simulink model "dc_motor"  (R2015a)
settings: Solver=ode45  StartTime=0.0  StopTime=0.3  RelTol=1e-3
values from neighbouring files (symbols this model uses):
  j = 0.575/1000    (= 0.000575)    [motor_a2b_param.m]    (also in motor_param.m = 0.02)
  k = 0.93    [motor_a2b_param.m]    (also in motor_param.m = 0.796; para.m = 0.5)
  la = 25/1000    (= 0.025)    [motor_a2b_param.m]    (also in motor_param.m = 0.01)
  ra = 7.8    [motor_a2b_param.m]    (also in motor_param.m = 0.78)
libraries: powerlib x5
settings Model: Creator=Windows 10  LastModifiedBy=Windows 10

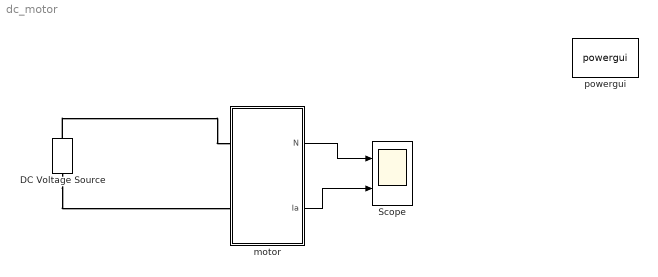
== system dc_motor ==
  DC Voltage Source : powerlib/Electrical Sources/DC Voltage Source  Amplitude=150  Measurements=None
  Scope : Scope  NumInputPorts=2
      settings: YMin=-5~-5  YMax=5~5
  "motor " : Subsystem
  powergui : powerlib/powergui  Priority=1  SimulationMode=Continuous  SolverType=Tustin/Backward Euler (TBE)  SampleTime=50e-6  frequency=60  SPID=off  DisableSnubberDevices=off  DisableRonSwitches=off  DisableVfSwitches=off  SwTol=0  DisplayEquations=off  Interpol=off  methode=off  Ts=100  FunctionMessages=off  echomessages=off  HookPort=off  EnableUseOfTLC=off  x0status=blocks  frequencyindice=0  Pbase=100e6  ErrMax=1e-4  Iterations=50  UnitsV=kV  UnitsW=MW  buscounter=0  RestoreLinks=warning  ResistiveCurrentMeasurement=off  Frange=[0:2:500]  Ylog=off  Xlog=on  ShowGrid=off  save=off  variable=ZData  structure=0  ZoomFFT=off  StartTime=0.0  cycles=1  DisplayStyle=1  fundamental=60  FreqAxis=off  MaxFrequency=1000  frequencyindicesteady=1  RmsSteady=1  display=off
  wires:
  "motor "/2("Ia ") -> Scope/2
  "motor "/1(N) -> Scope/1
  connections:
  DC Voltage Source/RConn1 -- "motor "/LConn1
  DC Voltage Source/LConn1 -- "motor "/LConn2

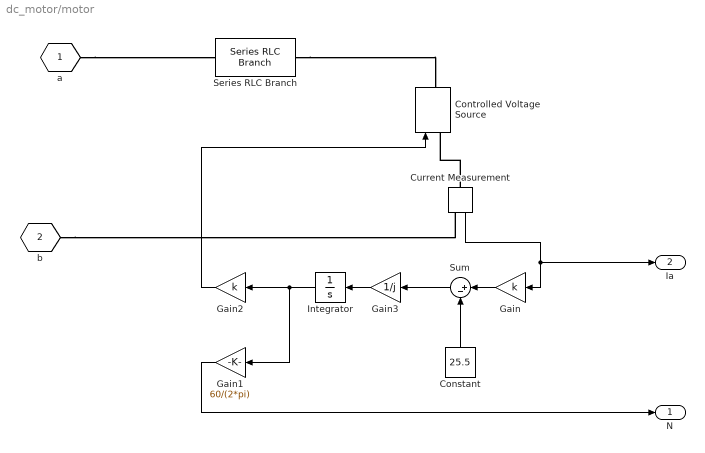
== system dc_motor/motor  ==
  Constant : Constant  Value=25.5
  Controlled Voltage Source : powerlib/Electrical Sources/Controlled Voltage Source  Initialize=on  Source_Type=AC  Amplitude=0  Phase=0  Frequency=0  Measurements=None
  Current Measurement : powerlib/Measurements/Current Measurement  PhasorSimulation=off  OutputType=Complex  PSBequivalent=0
  Gain : Gain  Gain=k
  Gain1 : Gain  Gain=60/(2*pi)
  Gain2 : Gain  Gain=k
  Gain3 : Gain  Gain=1/j
  Integrator : Integrator
  Series RLC Branch : powerlib/Elements/Series RLC Branch  LConnTagsString=__new0  RConnTagsString=__new0  BranchType=RL  Resistance=ra  Inductance=la  SetiL0=on  InitialCurrent=0  Capacitance=1e-6  Setx0=off  InitialVoltage=0  Measurements=None
  Sum : Sum  Inputs=|+-
  a : PMIOPort  Tag=PMCPort  Port=1  Side=Left
  b : PMIOPort  Tag=PMCPort  Port=2  Side=Left
  N : Outport
  "Ia " : Outport  Port=2
  wires:
  Current Measurement/1 -> "Ia "/1, Gain/1
  Gain/1 -> Sum/1
  Constant/1 -> Sum/2
  Sum/1 -> Gain3/1
  Gain3/1 -> Integrator/1
  Integrator/1 -> Gain1/1, Gain2/1
  Gain2/1 -> Controlled Voltage Source/1
  Gain1/1 -> N/1
  connections:
  a/RConn1 -- Series RLC Branch/LConn1
  Series RLC Branch/RConn1 -- Controlled Voltage Source/RConn1
  Current Measurement/LConn1 -- Controlled Voltage Source/LConn1
  b/RConn1 -- Current Measurement/RConn1
